simulink model "car_pendulum_control_with_observer"  (R2020b)
settings: Solver=VariableStepAuto  StartTime=0.0  StopTime=6  FixedStep=0.001  RelTol=1e-3
settings Model: Creator=petir  LastModifiedBy=petir

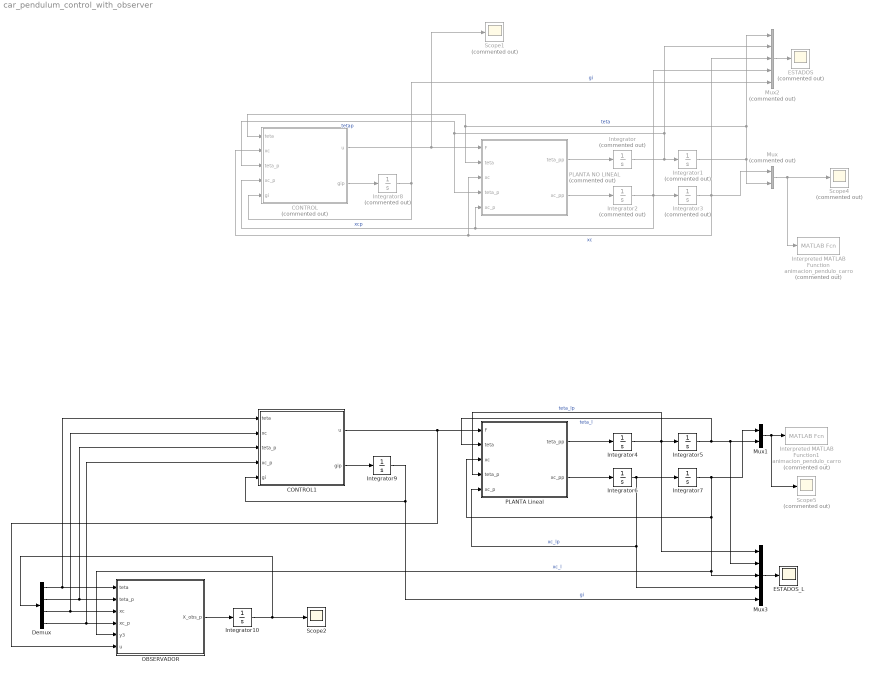
== system car_pendulum_control_with_observer ==
  CONTROL : MATLAB Function  Commented=on  TreatAsAtomicUnit=on
  CONTROL1 : MATLAB Function  TreatAsAtomicUnit=on
  Demux : Demux
  ESTADOS : Scope  Commented=on
  ESTADOS_L : Scope
  Integrator{,1..3,8} (5 alike) : Integrator  Commented=on
  Integrator10 : Integrator  InitialCondition=[0;0;0;0]
  Integrator{4..7,9} (5 alike) : Integrator
  Interpreted MATLAB Function : MATLABFcn  Commented=on  MATLABFcn=animacion_pendulo_carro  OutputDimensions=0
  Interpreted MATLAB Function1 : MATLABFcn  Commented=on  MATLABFcn=animacion_pendulo_carro  OutputDimensions=0
  Mux : Mux  Commented=on  Inputs=2
  Mux1 : Mux  Inputs=2
  Mux2 : Mux  Commented=on  Inputs=5
  Mux3 : Mux  Inputs=5
  OBSERVADOR : MATLAB Function  TreatAsAtomicUnit=on
  PLANTA Lineal : MATLAB Function  TreatAsAtomicUnit=on
  PLANTA NO LINEAL : MATLAB Function  Commented=on  TreatAsAtomicUnit=on
  Scope1 : Scope  Commented=on
  Scope2 : Scope
  Scope4 : Scope  Commented=on
  Scope5 : Scope  Commented=on
  wires:
  PLANTA NO LINEAL/1(teta_pp) -> Integrator/1
  Integrator/1 -> PLANTA NO LINEAL/4(teta_p), CONTROL/3(teta_p), Mux2/2, Integrator1/1  "tetap"
  Integrator1/1 -> Mux2/1, PLANTA NO LINEAL/2(teta), CONTROL/1(teta), Mux/2  "teta"
  PLANTA NO LINEAL/2(xc_pp) -> Integrator2/1
  Integrator2/1 -> CONTROL/4(xc_p), PLANTA NO LINEAL/5(xc_p), Mux2/4, Integrator3/1  "xcp"
  Integrator3/1 -> CONTROL/2(xc), PLANTA NO LINEAL/3(xc), Mux2/3, Mux/1  "xc"
  Integrator6/1 -> Integrator7/1, Mux3/4, PLANTA Lineal/5(xc_p)  "xc_lp"
  Integrator4/1 -> Integrator5/1, Mux3/1, PLANTA Lineal/4(teta_p)  "teta_lp"
  Integrator5/1 -> Mux3/2, Mux1/2, PLANTA Lineal/2(teta)  "teta_l"
  Integrator7/1 -> OBSERVADOR/5(y3), Mux3/3, PLANTA Lineal/3(xc), Mux1/1  "xc_l"
  PLANTA Lineal/1(teta_pp) -> Integrator4/1
  Mux/1 -> Scope4/1, Interpreted MATLAB Function/1
  Mux1/1 -> Scope5/1, Interpreted MATLAB Function1/1
  CONTROL/2(gip) -> Integrator8/1
  Integrator8/1 -> CONTROL/5(gi), Mux2/5  "gi"
  Mux2/1 -> ESTADOS/1
  CONTROL1/2(gip) -> Integrator9/1
  Integrator9/1 -> Mux3/5, CONTROL1/5(gi)  "gi"
  CONTROL1/1(u) -> OBSERVADOR/6(u), PLANTA Lineal/1(F)
  Mux3/1 -> ESTADOS_L/1
  CONTROL/1(u) -> Scope1/1, PLANTA NO LINEAL/1(F)
  OBSERVADOR/1(X_obs_p) -> Integrator10/1
  Integrator10/1 -> Demux/1, Scope2/1
  Demux/1 -> CONTROL1/1(teta), OBSERVADOR/1(teta)
  Demux/2 -> CONTROL1/3(teta_p), OBSERVADOR/2(teta_p)
  Demux/3 -> CONTROL1/2(xc), OBSERVADOR/3(xc)
  Demux/4 -> CONTROL1/4(xc_p), OBSERVADOR/4(xc_p)
  PLANTA Lineal/2(xc_pp) -> Integrator6/1

== matlab function car_pendulum_control_with_observer/PLANTA Lineal ==
  data: F input; teta_pp output; teta input; xc input; teta_p input; xc_p input; xc_pp output
function [teta_pp,xc_pp] = fcn(F, teta, xc, teta_p, xc_p)
m = 0.1;
M = 2;
l = 0.5;
L = 1;
g = 9.81;

% sin(teta) ~= 0
% xc_pp = F / (M + 2*m);
% teta_pp = -F / (l * (M + 2*m));

% sin(teta) ~= teta
% xc_pp = (F - m * g * teta) / M;
% teta_pp = (-F + (M + m) * g * teta) / M;

A = [0, 1, 0, 0; 
    (M+m)*g/(M*l), 0, 0, 0; 
    0, 0, 0, 1; 
    -m*g/M, 0, 0, 0];
B=[0; -1/(M*l); 0;  1/M];
X = [teta; teta_p; xc; xc_p];
salida = A*X + B*F;
teta_pp = salida(2);
xc_pp = salida(4);

== matlab function car_pendulum_control_with_observer/PLANTA NO LINEAL ==
  data: F input; teta_pp output; teta input; xc input; teta_p input; xc_p input; xc_pp output
function [teta_pp, xc_pp] = fcn(F, teta, xc, teta_p, xc_p)
m = 1;
M = 2;
l = 0.5;
L = 1;
g = 9.81;

det = ((M + m)*m*l^2 - (m*l*cos(teta))^2);

xc_pp = (m*l^2 * (F + m*l*sin(teta) * teta_p^2)... 
            - m*l*cos(teta) * (m*g*l*sin(teta))) / det;
teta_pp = (-m*l*cos(teta) * (F + m*l*sin(teta) * teta_p^2)...
            + (M + m)*(m*g*l*sin(teta))) / det;

== matlab function car_pendulum_control_with_observer/CONTROL ==
  data: teta input; xc input; teta_p input; xc_p input; gi input; u output; gip output
function [u, gip] = fcn(teta, xc, teta_p, xc_p, gi)
% Plant
M = 2;
m = 0.1; 
L = 0.5;
g = 9.81;
% Reference
r = 1;

A = [0 , 1, 0, 0; 
    (M+m)*g/(M*L), 0, 0, 0;
    0, 0, 0, 1;
    -m*g/M, 0, 0, 0];
B = [0; -1/(M*L); 0; 1/M];
C = [0, 0, 1, 0];

K = [-157.633619775739,-35.3733027419025,-56.0652395514781,-36.7466054838049];
Ki = -50.968399592252790;

% AA = [A-B*K, B*Ki; -C, 0];
% BB = [0; 0; 0; 0; 1];
% CC = [C 0];
% DD = [0]

X = [teta; teta_p; xc; xc_p];
Y = C * X;

u = -K * X + Ki*gi;
gip = r - Y;

== matlab function car_pendulum_control_with_observer/CONTROL1 ==
  data: teta input; xc input; teta_p input; xc_p input; gi input; u output; gip output
function [u, gip] = fcn(teta, xc, teta_p, xc_p, gi)
% Plant
M = 2;
m = 0.1; 
L = 0.5;
g = 9.81;
% Reference
r = 1;

A = [0 , 1, 0, 0; 
    (M+m)*g/(M*L), 0, 0, 0;
    0, 0, 0, 1;
    -m*g/M, 0, 0, 0];
B = [0; -1/(M*L); 0; 1/M];
C = [0, 0, 1, 0];

K = [-157.633619775739,-35.3733027419025,-56.0652395514781,-36.7466054838049];
Ki = -50.968399592252790;

% AA = [A-B*K, B*Ki; -C, 0];
% BB = [0; 0; 0; 0; 1];
% CC = [C 0];
% DD = [0]

X = [teta; teta_p; xc; xc_p];
Y = C * X;

u = -K * X + Ki * gi;
gip = r - Y;

== matlab function car_pendulum_control_with_observer/OBSERVADOR ==
  data: teta input; teta_p input; xc input; xc_p input; y3 input; u input; X_obs_p output
function X_obs_p = fcn(teta, teta_p, xc, xc_p, y3, u)
% Plant
M = 2;
m = 0.1; 
L = 0.5;
g = 9.81;
A = [0 , 1, 0, 0; 
    (M+m)*g/(M*L), 0, 0, 0;
    0, 0, 0, 1;
    -m*g/M, 0, 0, 0];
B = [0; -1/(M*L); 0; 1/M];
C = [0, 0, 1, 0];
Ke = [-4431.1; -633.4; -6371; -1146.8];
X_obs = [teta; teta_p; xc; xc_p];
% This is the output of the plant. y3 is the actual car speed.
% Y = C * [0, 0, y3, 0]';
% X_obs_p = (A - Ke*C) * X_obs + B * u + Ke*Y;
X_obs_p = A * X_obs + B * u + Ke * (y3 - C*X_obs);
